simulink model "project"  (R2015a)
settings: Solver=ode45  StartTime=0.0  StopTime=40  RelTol=1e-3
values from neighbouring files (symbols this model uses):
  A = [0 1 0 0 ... (first row only)    [task.m]
  B = [0 ... (first row only)    [task.m]
  C = [1 0 0 0]    [task.m]
  K = place(A, B, desired_controller_poles)    [task.m]
  L = place(A', C', desired_observer_poles)'    [task.m]
libraries: cstblocks x5, simulink x1
settings Model: Creator=saadc  LastModifiedBy=saadc

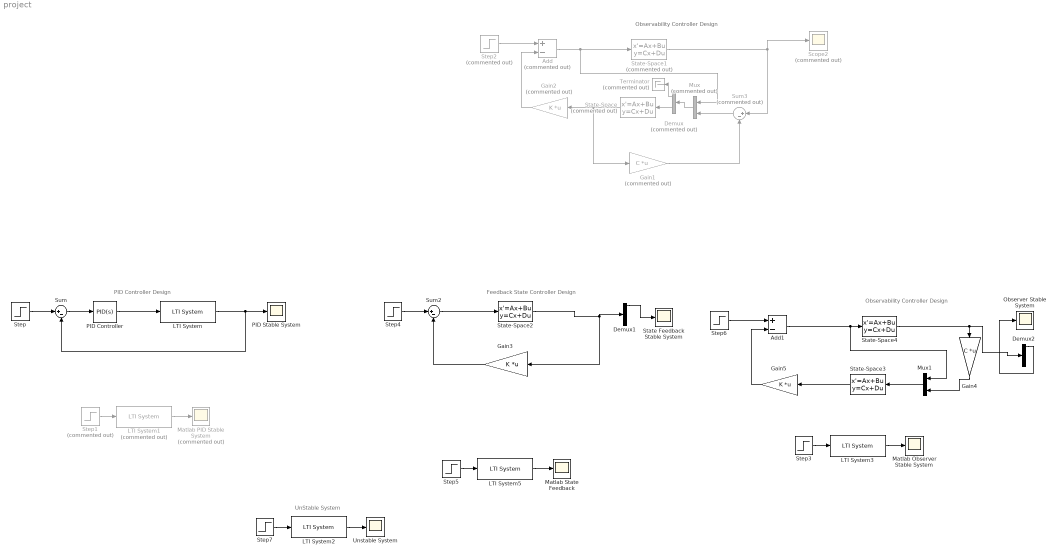
== system project ==
  note: PID Controller Design
  note: Feedback State Controller Design
  note: Observability Controller Design
  note: UnStable System
  note: Observability Controller Design
  Add : Sum  Commented=on  Inputs=+-
  Add1 : Sum  Inputs=+-
  Demux : Demux  Commented=on  Outputs=2
  Demux1 : Demux
  Demux2 : Demux
  Gain1 : Gain  Commented=on  Gain=C  Multiplication=Matrix(K*u)
  Gain2 : Gain  Commented=on  Gain=K  Multiplication=Matrix(K*u)
  Gain3 : Gain  Gain=K  Multiplication=Matrix(K*u)
  Gain4 : Gain  Gain=C  Multiplication=Matrix(K*u)
  Gain5 : Gain  Gain=K  Multiplication=Matrix(K*u)
  LTI System : cstblocks/LTI System  sys=sys_unstable  IC=[]
  LTI System1 : cstblocks/LTI System  Commented=on  sys=sys_cl_pid  IC=[]
  LTI System2 : cstblocks/LTI System  sys=sys_unstable  IC=[]
  LTI System3 : cstblocks/LTI System  sys=sys_observer_controller  IC=[]
  LTI System5 : cstblocks/LTI System  sys=sys_feedback_controller  IC=[]
  Matlab Observer Stable System : Scope
      settings: SaveName=ScopeData3
  Matlab PID Stable System : Scope  Commented=on
      settings: TimeRange=10  YMin=0  YMax=52.5
  Matlab State Feedback : Scope
      settings: YMin=2.5e-05  YMax=6.25e-05  SaveName=ScopeData5
  Mux : Mux  Commented=on  Inputs=2
  Mux1 : Mux  Inputs=2
  Observer Stable System : Scope
      settings: SaveName=ScopeData6
  PID Controller : simulink/Continuous/PID Controller  Controller=PID  TimeDomain=Continuous-time  SampleTime=-1  IntegratorMethod=Forward Euler  FilterMethod=Forward Euler  Form=Parallel  UseFilter=on  ControllerParametersSource=internal  P=-0.0552  I=-0.000684  D=-1.11  N=0  InitialConditionSource=internal  InitialConditionForIntegrator=0  InitialConditionForFilter=0  ExternalReset=none  LimitOutput=off  UpperSaturationLimit=inf  LowerSaturationLimit=-inf  LinearizeAsGain=on  AntiWindupMode=none  Kb=1  TrackingMode=off  Kt=1  PParamMin=[]  PParamMax=[]  IParamMin=[]  IParamMax=[]  DParamMin=[]  DParamMax=[]  NParamMin=[]  NParamMax=[]  KbParamMin=[]  KbParamMax=[]  KtParamMin=[]  KtParamMax=[]  POutMin=[]  POutMax=[]  IOutMin=[]  IOutMax=[]  DOutMin=[]  DOutMax=[]  NOutMin=[]  NOutMax=[]  KbOutMin=[]  KbOutMax=[]  KtOutMin=[]  KtOutMax=[]  IntegratorOutMin=[]  IntegratorOutMax=[]  FilterOutMin=[]  FilterOutMax=[]  SumOutMin=[]  SumOutMax=[]  SumI1OutMin=[]  SumI1OutMax=[]  SumI2OutMin=[]  SumI2OutMax=[]  SumI3OutMin=[]  SumI3OutMax=[]  SumDOutMin=[]  SumDOutMax=[]  SaturationOutMin=[]  SaturationOutMax=[]  IntegratorContinuousStateAttributes=''  IntegratorStateMustResolveToSignalObject=off  IntegratorRTWStateStorageClass=Auto  FilterContinuousStateAttributes=''  FilterStateMustResolveToSignalObject=off  FilterRTWStateStorageClass=Auto  DifferentiatorICPrevScaledInput=0  DifferentiatorOutMin=[]  DifferentiatorOutMax=[]
  PID Stable System : Scope
      settings: TimeRange=1  YMin=-10000000  YMax=140000000
  Scope2 : Scope  Commented=on
      settings: SaveName=ScopeData2
  State Feedback Stable System : Scope
      settings: TimeRange=40  YMin=-0.2325  YMax=-0.185  SaveName=ScopeData4
  State-Space : StateSpace  Commented=on  A=A-L*C  B=[B L]  C=eye(4)  D=[0 0;0 0;0 0;0 0]  X0=0
  State-Space1 : StateSpace  Commented=on  A=A  B=B  C=eye(4)  D=[0;0;0;0]  X0=0
  State-Space2 : StateSpace  A=A  B=B  C=eye(4)  D=[0;0;0;0]  X0=0
  State-Space3 : StateSpace  A=A-L*C  B=[B L]  C=eye(4)  D=[0 0;0 0;0 0;0 0]  X0=0
  State-Space4 : StateSpace  A=A  B=B  C=eye(4)  D=[0;0;0;0]  X0=0
  Step{,3..7} (6 alike) : Step  SampleTime=0
  Step1 : Step  Commented=on  SampleTime=0
  Step2 : Step  Commented=on  SampleTime=0
  Sum : Sum  Inputs=|+-
  Sum2 : Sum  Inputs=|+-
  Sum3 : Sum  Commented=on  Inputs=|+-
  Terminator : Terminator  Commented=on
  Unstable System : Scope
      settings: SaveName=ScopeData7
  wires:
  Sum/1 -> PID Controller/1
  PID Controller/1 -> LTI System/1
  Step/1 -> Sum/1
  LTI System/1 -> Sum/2, PID Stable System/1
  Step1/1 -> LTI System1/1
  LTI System1/1 -> Matlab PID Stable System/1
  Sum2/1 -> State-Space2/1
  Step4/1 -> Sum2/1
  Step5/1 -> LTI System5/1
  LTI System5/1 -> Matlab State Feedback/1
  Step3/1 -> LTI System3/1
  LTI System3/1 -> Matlab Observer Stable System/1
  Gain3/1 -> Sum2/2
  Add1/1 -> State-Space4/1, Mux1/1
  Step6/1 -> Add1/1
  State-Space3/1 -> Gain5/1
  Gain5/1 -> Add1/2
  Mux1/1 -> State-Space3/1
  Gain4/1 -> Mux1/2
  State-Space4/1 -> Demux2/1, Gain4/1
  Step7/1 -> LTI System2/1
  LTI System2/1 -> Unstable System/1
  Add/1 -> State-Space1/1, Mux/1
  Step2/1 -> Add/1
  Sum3/1 -> Mux/2
  State-Space/1 -> Gain1/1, Gain2/1
  Gain1/1 -> Sum3/2
  Gain2/1 -> Add/2
  Mux/1 -> Demux/1
  Demux/2 -> State-Space/1
  State-Space1/1 -> Scope2/1, Sum3/1
  Demux/1 -> Terminator/1
  State-Space2/1 -> Gain3/1, Demux1/1
  Demux1/1 -> State Feedback Stable System/1
  Demux2/1 -> Observer Stable System/1
